simulink model "Assignment_CellModel"  (R2019b)
settings: Solver=VariableStepAuto  StartTime=0.0  StopTime=900  MaxStep=0.01  RelTol=1e-3
settings Model: Creator=jorge  LastModifiedBy=jorge

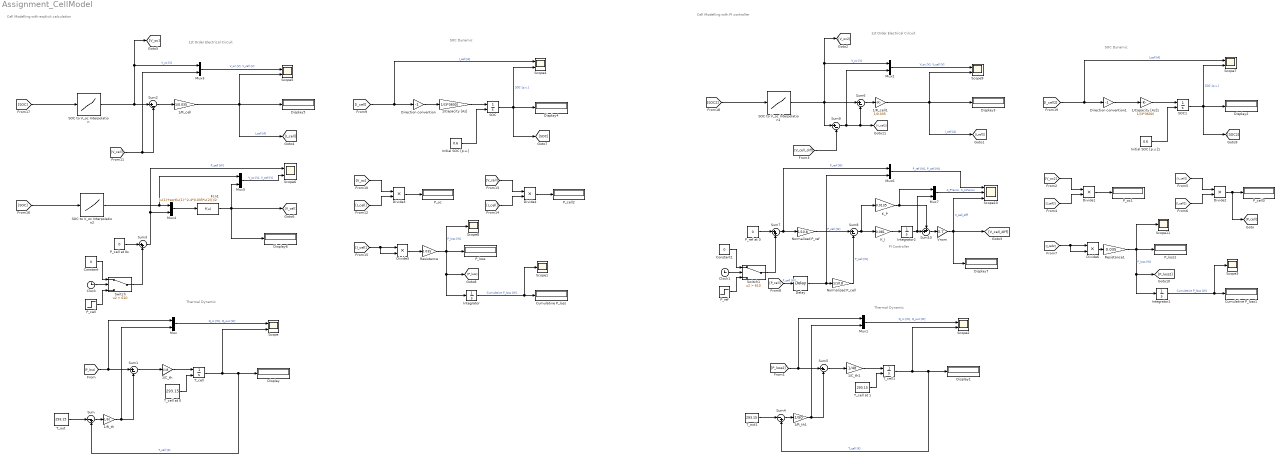
== system Assignment_CellModel ==
  note: PI Controller
  note: Thermal Dynamic
  note: SOC Dynamic
  note: 1st Order Electrical Circuit
  note: 1st Order Electrical Circuit
  note: Thermal Dynamic
  note: SOC Dynamic
  note: Cell Modelling with explicit calculation
  note: Cell Modelling with PI controller
  1/C_th : Gain  Gain=1/48
  1/C_th1 : Gain  Gain=1/48
  1/Capacity [As] : Gain  Gain=1/(3*3600)
  1/Capacity [As]1 : Gain  Gain=1/(3*3600)
  1/R_cell : Gain  Gain=1/0.035
  1/R_cell1 : Gain  Gain=1/0.035
  1/R_th : Gain  Gain=1/50
  1/R_th1 : Gain  Gain=1/50
  Clock : Clock
  Clock1 : Clock
  Constant : Constant  Value=0
  Constant1 : Constant  Value=0
  Cumulative P_loss : Display
  Cumulative P_loss1 : Display
  Delay : TransportDelay  DelayTime=0.1
  Direction convention : Gain  Gain=-1
  Direction convention1 : Gain  Gain=-1
  Display{,1..7} (8 alike) : Display
  Divide{1..6} (6 alike) : Product  Inputs=**
  Fcn1 : Fcn  Expr=(u(1)+sqrt(u(1)^2-4*0.035*u(2)))/2
  Initial SOC [p.u.] : Constant  Value=0.6
  Initial SOC [p.u.]1 : Constant  Value=0.6
  Integrator : Integrator
  Integrator1 : Integrator
  Integrator2 : Integrator
  K_I : Gain  Gain=0.081
  K_P : Gain  Gain=0.0135
  Mux{,1..7} (8 alike) : Mux  Inputs=2
  Normalized P_cell : Gain  Gain=1/10.8
  Normalized P_ref : Gain  Gain=1/10.8
  P_cell : Step  Time=10  After=20  SampleTime=0
  P_cell at 0s : Constant  Value=0
  P_cell2 : Display
  P_cell3 : Display
  P_loss : Display
  P_loss1 : Display
  P_oc : Display
  P_oc1 : Display
  P_ref : Step  Time=10  After=20  SampleTime=0
  P_ref at 0 : Constant  Value=0
  Resistance : Gain  Gain=0.035
  Resistance1 : Gain  Gain=0.035
  SOC : Integrator  InitialConditionSource=external  InitialCondition=0.5
  SOC to V_oc Interpolation : Lookup_n-D  NumberOfTableDimensions=1  BreakpointsForDimension1=[0,0.1,0.2,0.3,0.4,0.5,0.6,0.7,0.8,0.9,1]  UseOneInputPortForAllInputData=on  Table=[2.85,3.19,3.39,3.52,3.65,3.73,3.82,3.92,4.01,4.07,4.19]  InternalRulePriority=Speed  RndMeth=Simplest  InputSameDT=on
  SOC to V_oc Interpolation1 : Lookup_n-D  NumberOfTableDimensions=1  BreakpointsForDimension1=[0,0.1,0.2,0.3,0.4,0.5,0.6,0.7,0.8,0.9,1]  UseOneInputPortForAllInputData=on  Table=[2.85,3.19,3.39,3.52,3.65,3.73,3.82,3.92,4.01,4.07,4.19]  InternalRulePriority=Speed  RndMeth=Simplest  InputSameDT=on
  SOC to V_oc Interpolation2 : Lookup_n-D  NumberOfTableDimensions=1  BreakpointsForDimension1=[0,0.1,0.2,0.3,0.4,0.5,0.6,0.7,0.8,0.9,1]  UseOneInputPortForAllInputData=on  Table=[2.85,3.19,3.39,3.52,3.65,3.73,3.82,3.92,4.01,4.07,4.19]  InternalRulePriority=Speed  RndMeth=Simplest  InputSameDT=on
  SOC1 : Integrator  InitialConditionSource=external  InitialCondition=0.5
  Scope{,2,4..7,9} (7 alike) : Scope  NumInputPorts=2
  Scope{1,3,8,11} (4 alike) : Scope
  Scope10 : Scope  NumInputPorts=3
  Sum : Sum  Inputs=|-+
  Sum{1..2,5..6,8..9} (6 alike) : Sum  Inputs=|+-
  Sum10 : Sum  Inputs=++|
  Sum3 : Sum  Inputs=|++
  Sum4 : Sum  Inputs=|-+
  Sum7 : Sum  Inputs=|++
  Switch : Switch  Criteria=u2 > Threshold  Threshold=610
  Switch1 : Switch  Criteria=u2 > Threshold  Threshold=610
  T_cell : Integrator  InitialConditionSource=external  InitialCondition=20
  T_cell at 0 : Constant  Value=293.15
  T_cell at 1 : Constant  Value=293.15
  T_cell1 : Integrator  InitialConditionSource=external  InitialCondition=20
  T_out : Constant  Value=293.15
  T_out1 : Constant  Value=293.15
  Vnom : Gain  Gain=3.7
  wires:
  Divide3/1 -> P_oc/1
  [V_oc] -> Divide3/1
  Mux4/1 -> Fcn1/1
  SOC to V_oc Interpolation2/1 -> Mux4/1, Mux5/1
  Mux3/1 -> Scope5/1  "V_oc [V], V_cell [V]"
  P_cell at 0s/1 -> Sum3/1
  [I_cell] -> Scope4/1, Direction convention/1  "I_cell [A]"
  [V_cell] -> Mux3/2, Sum2/2
  1/R_cell/1 -> Scope5/2, Display5/1, [I_cell]  "I_cell [A]"
  Sum2/1 -> 1/R_cell/1
  [I_cell] -> Divide5/2, Divide5/1
  SOC to V_oc Interpolation/1 -> [V_oc], Mux3/1, Sum2/1  "V_oc [V]"
  [SOC] -> SOC to V_oc Interpolation/1
  1/Capacity [As]/1 -> SOC/1
  SOC/1 -> [SOC], Scope4/2, Display4/1  "SOC [p.u.]"
  Initial SOC [p.u.]/1 -> SOC/2
  Direction convention/1 -> 1/Capacity [As]/1
  Fcn1/1 -> Display6/1, Mux5/2, [V_cell]
  Sum3/1 -> Mux4/2, Scope6/1  "P_cell [W]"
  [SOC] -> SOC to V_oc Interpolation2/1
  [I_cell] -> Divide4/2
  Divide4/1 -> P_cell2/1
  Divide5/1 -> Resistance/1
  [V_cell] -> Divide4/1
  Resistance/1 -> P_loss/1, Integrator/1, [P_loss], Scope8/1  "P_loss [W]"
  [I_cell] -> Divide3/2
  Mux5/1 -> Scope6/2  "V_oc [V], V_cell [V]"
  1/C_th/1 -> T_cell/1
  T_cell at 0/1 -> T_cell/2
  T_cell/1 -> Scope/2, Display/1, Sum/2  "T_cell [K]"
  T_out/1 -> Sum/1
  Sum/1 -> 1/R_th/1
  1/R_th/1 -> Mux/2, Sum1/2
  [P_loss] -> Mux/1, Sum1/1
  Sum1/1 -> 1/C_th/1
  Mux/1 -> Scope/1  "Q_in [W], Q_out [W]"
  Integrator/1 -> Scope1/1, Cumulative P_loss/1  "Cumulative P_loss [W]"
  Clock/1 -> Switch/2
  Switch/1 -> Sum3/2
  P_cell/1 -> Switch/3
  Constant/1 -> Switch/1
  Constant1/1 -> Switch1/1
  1/C_th1/1 -> T_cell1/1
  [I_cell2] -> Scope7/1, Direction convention1/1  "I_cell [A]"
  1/Capacity [As]1/1 -> SOC1/1
  Direction convention1/1 -> 1/Capacity [As]1/1
  1/R_th1/1 -> Mux1/2, Sum5/2
  P_ref/1 -> Switch1/3
  T_out1/1 -> Sum4/1
  [V_oc2] -> Divide1/1
  [I_cell2] -> Divide2/2
  Switch1/1 -> Sum7/2
  P_ref at 0/1 -> Sum7/1
  [SOC2] -> SOC to V_oc Interpolation1/1
  Integrator1/1 -> Scope3/1, Cumulative P_loss1/1  "Cumulative P_loss [W]"
  Sum4/1 -> 1/R_th1/1
  Clock1/1 -> Switch1/2
  SOC1/1 -> [SOC2], Scope7/2, Display2/1  "SOC [p.u.]"
  T_cell1/1 -> Scope2/2, Display1/1, Sum4/2  "T_cell [K]"
  [I_cell2] -> Divide1/2
  [P_loss2] -> Mux1/1, Sum5/1
  SOC to V_oc Interpolation1/1 -> Sum9/1, [V_oc2], Mux2/1, Sum6/1  "V_oc [V]"
  Divide6/1 -> Resistance1/1
  [V_cell2] -> Divide2/1
  T_cell at 1/1 -> T_cell1/2
  Divide2/1 -> [P_cell], P_cell3/1
  Resistance1/1 -> P_loss1/1, Integrator1/1, [P_loss2], Scope11/1  "P_loss [W]"
  Mux1/1 -> Scope2/1  "Q_in [W], Q_out [W]"
  Mux2/1 -> Scope9/1  "V_oc [V], V_cell [V]"
  Sum6/1 -> 1/R_cell1/1
  Initial SOC [p.u.]1/1 -> SOC1/2
  1/R_cell1/1 -> Scope9/2, Display3/1, [I_cell2]  "I_cell [A]"
  [I_cell2] -> Divide6/2, Divide6/1
  Divide1/1 -> P_oc1/1
  Sum5/1 -> 1/C_th1/1
  Sum8/1 -> K_P/1, K_I/1
  Normalized P_ref/1 -> Sum8/1
  Sum7/1 -> Mux6/1, Normalized P_ref/1  "P_ref [W]"
  Normalized P_cell/1 -> Sum8/2  "P_cell [W]"
  Delay/1 -> Mux6/2, Normalized P_cell/1  "P_cell [W]"
  [V_cell_diff] -> Sum9/2
  Sum9/1 -> Mux2/2, [V_cell2], Sum6/2
  Vnom/1 -> Scope10/3, Display7/1, [V_cell_diff]  "V_cell_diff"
  K_I/1 -> Integrator2/1
  K_P/1 -> Mux7/1, Sum10/1
  Integrator2/1 -> Mux7/2, Sum10/2
  Sum10/1 -> Vnom/1
  Mux7/1 -> Scope10/2  "K_P*error, K_I/s*error"
  Mux6/1 -> Scope10/1  "P_ref [W], P_cell [W]"
  [P_cell] -> Delay/1  "P_cell [W]"
